simulink model "mdlref_F2C"  (Simulink 6.0)
settings: Solver=FixedStepDiscrete  SolverMode=SingleTasking  StartTime=0.0  StopTime=2*24*60*60  FixedStep=60  RelTol=1e-3  AbsTol=1e-6
settings Model: Creator=The MathWorks Inc.  LastModifiedBy=batserve  ExtModeAutoUpdateStatusClock=off
settings DataIOCC: ExternalInput=[]  InitialState=[]  LimitDataPoints=off  SaveOutput=off  SaveTime=off
settings OptimizationCC: BlockReduction=off  BooleanDataType=off  InlineParams=on
settings DebuggingCC: CheckExecutionContextPreStartOutputMsg=on  CheckExecutionContextRuntimeOutputMsg=on  SignalResolutionControl=UseLocalSettings  SolverPrmCheckMsg=none  IntegerOverflowMsg=none
settings HardwareCC: TargetUnknown=on

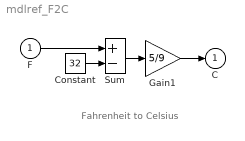
== system mdlref_F2C ==
  note: Fahrenheit to Celsius
  F : Inport  Port=1  PortDimensions=1  SampleTime=0  DataType=double  LatchInput=off
  Constant : Constant  Value=32
  Gain1 : Gain  Gain=5/9  SaturateOnIntegerOverflow=on
  Sum : Sum  Inputs=+-  SaturateOnIntegerOverflow=on  InputSameDT=on
  C : Outport  InitialOutput=0
  wires:
  Gain1/1 -> C/1
  Sum/1 -> Gain1/1
  F/1 -> Sum/1
  Constant/1 -> Sum/2
